simulink model "CANopen_CAN_Sender_Receiver"  (R2021b)
settings: Solver=VariableStepAuto  StartTime=0.0  StopTime=10.0  RelTol=1e-3
undefined symbols (not defined in the file): canChannel
libraries: simulink x48, commutil2 x5, canlib x3, dspindex x3, etargetslib x2, canmsglib x1
(part 2 of 2)

== stateflow chart CANopen_CAN_Sender_Receiver/Chart1 ==
  state Transreceive
    state Response [parallel]
      settings: executionOrder=3
      state Response_State [parallel]
        settings: executionOrder=1
        state Positive
          Enb=boolean(1);
          Abort_No(Req_Msg_No)=0;
          Delay_No(Req_Msg_No)=0;
          exit: Enb=boolean(0);
        state Abort
          Abort_No(Req_Msg_No)...
          =Abort_No(Req_Msg_No)+1;
          Abort=1;
          exit: Abort=0;
        state No_Req
          Enb=boolean(0);
        state Negative
          Res_steps(Res_Mes_Num)...
          =max(1,min(5,...
          (Req_Que(Res_Mes_Num)+...
          Delay_No(Res_Mes_Num))))
          Neg=1;
          exit: Neg=0;
        state Delay
          Delay=1;
          exit: Delay=0;
          (default) -> (junction 326)
          (junction 326) -> (junction 328) [order 1] : [NR==0]
              | {NR=1}
          (junction 326) -> (junction 330) [order 2] : {Delay_No(Req_Msg_No)...
              |     =Delay_No...
              |     (Req_Msg_No)+1;NR=0}
        state Error
          E=1;
        (junction 136) -> Abort [order 2] : [Res_Mes_Num==Req_Msg_No ...
            | &&Res_Abort==1&&Resp_Age==0]
        (default) -> (junction 136)
        (junction 136) -> Positive [order 3] : [Res_Mes_Num==Req_Msg_No&&...
            | Resp_Age==0&&(Res_Que(Res_Mes_Num)...
            | -Req_Que(Res_Mes_Num))<=1]
        (junction 136) -> Delay [order 5] : [Resp_Age>0&&(Req~=0||NR==1)&& ...
            | (Res_Mes_Num~=Req_Msg_No)]
        (junction 136) -> No_Req [order 6] : [Req==0]
        (junction 136) -> Negative [order 4] : [(Res_Mes_Num~=Req_Msg_No)&&...
            | (Req_Que(Res_Mes_Num)+Temp_Del...
            | >=Res_steps(Res_Mes_Num))&&Resp_Age==0]
        (junction 136) -> No_Req [order 1] : [Reset==1]
        (junction 136) -> Error [order 7]
      state Data_Store [parallel]
        settings: executionOrder=2
        (default) -> (junction 349)
        (junction 374) -> (junction 377) : {Vld_pass(1)=Last_cmd(1)- ...
            | Saved_Data(Res_Mes_Num)<1}
        (junction 357) -> (junction 374) [order 1] : [Res_Mes_Num==1]
        (junction 377) -> (junction 383)
        (junction 349) -> (junction 355) [order 1] : [Res_Mes_Num==15||Res_Mes_Num==16 ...
            | || Res_Mes_Num==17]
        (junction 349) -> (junction 359) [order 2]
        (junction 355) -> (junction 357)
        (junction 359) -> (junction 357) [order 1] : [Enb==1]{Saved_Data(Res_Mes_Num)=...
            | Res_Act_Data,Res_State(Res_Mes_Num)=1}
        (junction 357) -> (junction 379) [order 2] : [Res_Mes_Num==2]
        (junction 357) -> (junction 381) [order 3] : [Res_Mes_Num==3]
        (junction 359) -> (junction 364) [order 2]
        (junction 357) -> (junction 362) [order 4]
        (junction 379) -> (junction 383) : {Vld_pass(2)=Last_cmd(2)- ...
            | Saved_Data(Res_Mes_Num)<1}
        (junction 383) -> (junction 385)
        (junction 364) -> (junction 362) [order 1] : [(Abort==1&&Abort_No(Req_Msg_No)>2)||(Delay==1&&...
            | Delay_No(Req_Msg_No)>Res_steps(Req_Msg_No))]
            | {Saved_Data(Res_Mes_Num)=...
            | Default(Res_Mes_Num),Res_State(Res_Mes_Num)=-1}
        (junction 364) -> (junction 369) [order 2]
        (junction 362) -> (junction 367)
        (junction 381) -> (junction 385) : {Vld_pass(3)=Last_cmd(3)- ...
            | Saved_Data(Res_Mes_Num)<1}
        (junction 385) -> (junction 403)
        (junction 369) -> (junction 367) [order 1] : [~Reset]{Saved_Data(Req_Msg_No)=Saved_Data...
            | (Req_Msg_No),Res_State(Res_Mes_Num)=0}
        (junction 369) -> (junction 398) [order 2]
        (junction 367) -> (junction 400)
        (junction 398) -> (junction 400)
        (junction 403) -> (junction 400)
    state Request [parallel]
      settings: executionOrder=4
      state [Q_Data,Q_mNo,Com_Set] = Imp_Req ... [function]
        (Command_Throttle,Command_Brake, ...
        Command_Steer,SD)
      state [Q_Data,Q_mNo,Com_Set] = Other_Req(omit) [function]
      state [Q_Data,Q_mNo,Com_Set] = Logic_Based [function]
      (default) -> (junction 195) : {Req=1;superdelay=boolean(0);}
      (junction 211) -> (junction 233) [order 1] : [Set==5]
      (junction 195) -> (junction 211) [order 3] : [Reset||Enb==boolean(1)]{Cnt_Neg=0}
      (junction 288) -> (junction 211) : {omit(Req_Msg_No)=omit(Req_Msg_No)+1}
      (junction 233) -> (junction 214) : [Derate==1 ...
          | && Res_Que(15)<5]...
          | {[Req_Data_Act,Req_Msg_No,...
          | Set]=Logic_Based}
      (junction 211) -> (junction 214) [order 2] : [Res_Mes_Num==4||omit(4)>...
          | omit_p&& Res_Que(15)<10]...
          | {omit_p=omit(4),...
          | [Req_Data_Act,Req_Msg_No,...
          | Set]=Other_Req(omit)}
      (junction 195) -> (junction 228) [order 1] : [(Res_steps(15) ...
          | + Res_steps(16) ...
          | + Res_steps(17)...
          | +Res_steps(4))>40]...
          | {superdelay=boolean(1),...
          | [Req_Data_Act,...
          | Req_Msg_No,Set]=...
          | Imp_Req(VCL_Thr...
          | ,VCL_Brk,VCL_Str,superdelay)}
      (junction 195) -> (junction 209) [order 2] : [Set==1]
          | {Req=0;
          | Set=5;}
      (junction 211) -> (junction 214) [order 3] : {[Req_Data_Act,...
          | Req_Msg_No,Set]=...
          | Imp_Req(VCL_Thr...
          | ,VCL_Brk,VCL_Str,...
          | superdelay)}
      (junction 195) -> (junction 207) [order 4]
      (junction 218) -> (junction 288) [order 2] : {Abort_No(Req_Msg_No)=0}
      (junction 213) -> (junction 288) [order 2] : {Temp_Del=Delay_No(Req_Msg_No),
          | Delay_No(Req_Msg_No)=0}
      (junction 207) -> (junction 218) [order 1] : [Abort==1]
          | {Cnt_Neg=0}
      (junction 218) -> (junction 215) [order 1] : [Abort_No(Req_Msg_No)>=1 ...
          | && Abort_No(Req_Msg_No)<3]
      (junction 222) -> (junction 215)
      (junction 207) -> (junction 209) [order 2] : [NR==1]
          | {Req=0;}
      (junction 215) -> (junction 214) : {Req_Msg_No=...
          | Req_Msg_No}
      (junction 207) -> (junction 208) [order 3]
      (junction 208) -> (junction 213) [order 1] : [Delay==1]
          | {Cnt_Neg=0}
      (junction 213) -> (junction 222) [order 1] : [Delay_No(Req_Msg_No)>=1 ...
          | && Delay_No(Req_Msg_No)<...
          | Res_steps(Req_Msg_No)]
      (junction 208) -> (junction 295) [order 2]
      (junction 295) -> (junction 297) [order 1] : [Neg==1]
      (junction 297) -> (junction 222) : {Cnt_Neg = Cnt_Neg + 1}
      (junction 295) -> (junction 209) [order 2] : {Req=0;}
      (junction 214) -> (junction 209) [order 4]
      (junction 310) -> (junction 209) : {Last_cmd(1)=VCL_Thr}
      (junction 214) -> (junction 310) [order 1] : [Req_Msg_No==15]
      (junction 214) -> (junction 313) [order 2] : [Req_Msg_No==16]
      (junction 313) -> (junction 209) : {Last_cmd(2)=VCL_Brk}
      (junction 214) -> (junction 316) [order 3] : [Req_Msg_No==17]
      (junction 316) -> (junction 209) : {Last_cmd(3)=VCL_Str}
      (junction 209) -> (junction 212)
      (junction 228) -> (junction 212)
    state Queue_Update [parallel]
      settings: executionOrder=2
      (default) -> (junction 158)
      (junction 158) -> (junction 159) [order 1] : [~Reset]{Q_QueP=Req_Que, ...
          | S_QueP=Res_Que,[Res_Que, Req_Que] = ...
          | Queue(Req_Msg_No,...
          |  Res_Mes_Num, Q_QueP, S_QueP,...
          | Req, Resp_Age)}
      (junction 158) -> (junction 161) [order 2] : {Res_Que=zeros(17,1)...
          | ,Req_Que=zeros(17,1)}
    state Identifying_Message [parallel]
      settings: executionOrder=1
      state [Mes_No,Act_Data,Seg_Req,Abort] = Disintegrate(Data) [function]
      (junction 391) -> (junction 393) [order 1] : [Reset==1]
      (default) -> (junction 391)
      (junction 391) -> (junction 395) [order 2] : {[Res_Mes_Num,Res_Act_Data,Res_Seg_Req,Res_Abort]=...
          |     Disintegrate(Resp_Data);}
    state Requesting_Message [parallel]
      settings: executionOrder=5
      state [Raw_Data,Raw_Len] = Integrate(Req_Msg,Data) [function]
      (default) -> (junction 57)
      (junction 57) -> (junction 58) [order 1] : [Req==1]{[Req_Data,Req_Len]=...
          |     Integrate(Req_Msg_No,Req_Data_Act)}
      (junction 58) -> (junction 61)
      (junction 57) -> (junction 61) [order 2]
      (junction 61) -> (junction 413) : {Wait=1}
  state No_SDO_Comm
  state Wait [commented out]
    en:
    Tmr_W=1, Wait=0;
    du:
    Tmr_W = Tmr_W + 1
  (default) -> No_SDO_Comm
  Transreceive -> No_SDO_Comm [order 1] : [Abort_No(15)==2||...
      | Abort_No(16)==2||...
      | Abort_No(17)==2||...
      | Cnt_Neg>=3]{Fault=1}
  No_SDO_Comm -> Transreceive : [Res==1]{Reset=1}
  Transreceive -> (junction 418) [order 2] : [Wait==1]
      | {Wait=0}
  (junction 418) -> Transreceive [order 2] : {Reset=0}
  (junction 418) -> Transreceive [order 1] : [~Fir_Mes]
      | {Reset=1}
  Wait -> Transreceive [commented out] : [Tmr_W>=1]{Tmr_W=0}
  data: Command_Throttle function_input int8 size=1; Command_Brake function_input int8 size=1; Command_Steer function_input int8 size=1; Q_Data function_output uint16; Q_mNo function_output uint8; Com_Set function_output; SD function_input boolean size=1; Q_Data function_output uint16; Q_mNo function_output uint8; omit function_input uint8 size=17; Com_Set function_output; Q_Data function_output uint16; Q_mNo function_output uint8; Com_Set function_output; S_Que function_output size=17; Q_Que function_output; Q_Msg_No function_input; S_Mes_Num function_input; Q_QuePrevious function_input; S_QuePrevious function_input; Req_High function_input; Age function_input; Data function_input uint8 size=8; Mes_No function_output uint8; Act_Data function_output; Seg_Req function_output boolean; Abort function_output uint8; Raw_Data function_output; Req_Msg function_input uint8 size=1; Data function_input uint16 size=1; Raw_Len function_output; Resp_Age input; Resp_DLC_bool input; Resp_Data input size=8; Res_Mes_Num local uint8 =uint8(0); Res_Act_Data local double; Res_Seg_Req local boolean; Req_Data output size=8; Req_Len output size=1; Req_Data_Act local uint16 size=1; Req_Msg_No local uint8 size=1 =uint8(0); Req local; VCL_Thr input int8; VCL_Brk input int8; VCL_Str input int8; Res_Abort local; Abort_No output =zeros(17,1); Delay_No output size=17 =zeros(17,1); Fault output =0; omit output uint8 size=17 =uint8(zeros(17,1)); Res_steps local =2*ones(17,1); Abort local =0; Delay local =0; Set local =0; E output =0; Q_QueP local; S_QueP local; Enb output boolean size=1; omit_p local =uint8(0); Derate input; Neg local =0; Req_Que local; Res_Que local; superdelay local boolean; Cnt_Neg local =0; Last_cmd output size=3 =zeros(3,1); NR local =0; Res_State output =ones(17,1); Saved_Data output =zeros(17,1); Default input; Vld_pass output =boolean(ones(3,1)); Res input; Reset local; Tmr_W local; Wait local; Temp_Del local =0; Fir_Mes input
  function [S_Que, Q_Que] = Queue(Q_Msg_No, S_Mes_Num...:
    | function [S_Que, Q_Que] = Queue(Q_Msg_No, S_Mes_Num...
    |     , Q_QuePrevious, S_QuePrevious,Req_High, Age)
    | 
    | % Queue1(Res_Mes_Num,QueP)
    | % Queue2(Req_Msg_No,QueP)
    | 
    | 
    | Q_Que=zeros(17,1);
    | Q_Que(:)=Q_QuePrevious(:)+1;
    | 
    | if Req_High==1
    | Q_Que(Q_Msg_No)=0;
    | end
    | 
    | S_Que=zeros(17,1);
    | S_Que(:)=S_QuePrevious(:)+1;
    | 
    | if Age==0
    |     S_Que(S_Mes_Num)=0;
    | end
